simulink model "RO_Plantsimscape"  (R2020a)
settings: Solver=VariableStepAuto  StartTime=0.0  StopTime=100  RelTol=1e-3
libraries: sh_lib x108, fl_lib x76, nesl_utility x73, simulink x13
(part 2 of 4)

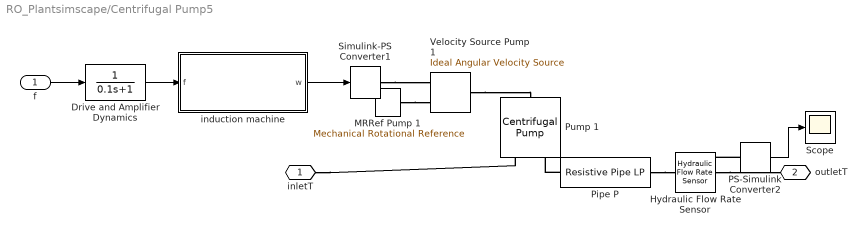
== system RO_Plantsimscape/Centrifugal Pump5 ==
  f : Inport
  Drive and Amplifier Dynamics : TransferFcn  Denominator=[0.1 1]
  Hydraulic Flow Rate Sensor : fl_lib/Hydraulic/Hydraulic Sensors/Hydraulic Flow Rate Sensor
  MRRef Pump 1 : fl_lib/Mechanical/Rotational Elements/Mechanical Rotational Reference
  PS-Simulink Converter2 : nesl_utility/PS-Simulink Converter  PhysicalDomain=network_engine_domain  SubClassName=ps_output  LeftPortType=input  RightPortType=output  PseudoPeriodic=off  Frequencies=[]  Unit=1  AffineConversion=off
  Pipe P : sh_lib/Low-Pressure Blocks/Resistive Pipe LP  cs_type=1  d_in=112.1660 mm  area=1e-04 m^2  D_h=0.0112 m  s_factor=64  length=8.1 m  length_ad=1 m  roughness=0.005 mm  Re_lam=2e+03  Re_turb=4e+03  elevation_A=45 m  elevation_B=45 m  g=9.80665 m/s^2  pressure_drop_specify=off  pressure_drop_priority=None  pressure_drop=0 Pa  pressure_drop_nominal_specify=off  pressure_drop_nominal_unit=Pa  pressure_drop_nominal_value=1  flow_rate_specify=off  flow_rate_priority=None  flow_rate=0 m^3/s  flow_rate_nominal_specify=off  flow_rate_nominal_unit=m^3/s  flow_rate_nominal_value=1
      settings: SourceProductBaseCode=SH  InternalSimscapePortConfiguration="{\"Bottom\":[],\"Left\":[{\"id\":\"A\",\"label\":\"A\",\"type\":\"foundation.hydraulic.hydraulic\"}],\"Right\":[{\"id\":\"B\",\"label\":\"B\",\"type\":\"foundation.hydraulic.hydraulic\"}],\"Top\":[]}"
  Pump 1 : sh_lib/Pumps and Motors/Centrifugal Pump  mdl_type=2  c_1=326.8 Pa/(kg/m^3)  c_2=3.104e+04 Pa*s/kg  c_3=1.097e+07 Pa*s^2/(kg*m^3)  c_4=2.136e+05 Pa*s^2/(kg*m^3)  c_f=0.8  design_del=130 lpm  ref_velocity=1.77e+03 rpm  ref_density=1000 kg/m^3  leak_resistance=1e+8 Pa/(m^3/s)  T_const=0.1 N*m  trq_press_coeff=1e-6 N*m/Pa  pump_del_1D="[0    0.0032    0.0063    0.0095    0.0126    0.0158] m^3/s"  press_diff_1D="[4.4851    4.3655    4.1413    3.7376    2.9901    1.7940] bar"  pump_del_power_1D="[0    0.0032    0.0063    0.0095    0.0126    0.0158] m^3/s"  power_1D="[0\t2116.60000000000\t3727.20000000000\t4734.30000000000\t5232.70000000000\t4360.90000000000] W"  pump_vel_2D="[  3.2e+03 3.3e+03 3.4e+03 3.5e+03 ] rpm"  pump_del_2D="[  0 50 100 150 200 250 300 350 ] lpm"  press_diff_2D="[  8.3 8.8 9.3 9.9 ; 7.8 8.3 8.8 9.4 ; 7.2 7.6 8.2 8.7 ; 6.5 7 7.5 8 ; 5.6 6.1 6.6 7.1 ; 4.7 5.2 5.7 6.2 ; 3.4 4 4.4 4.9 ; 2.3 2.7 3.4 3.6 ; ] bar"  pump_del_power_2D="[  0 50 100 150 200 250 300 350 ] lpm"  power_2D="[  1.223e+03 1.341e+03 1.467e+03 1.6e+03 ; 1.414e+03 1.551e+03 1.696e+03 1.85e+03 ; 1.636e+03 1.794e+03 1.962e+03 2.14e+03 ; 1.941e+03 2.129e+03 2.326e+03 2.54e+03 ; 2.224e+03 2.439e+03 2.66e+03 2.91e+03 ; 2.453e+03 2.691e+03 2.947e+03 3.21e+03 ; 2.757e+03 3.024e+03 3.307e+03 3.608e+03 ; 2.945e+03 3.23e+03 3.533e+03 3.854e+03 ; ] W"  omega_threshold=1e-9 rad/s  interp_method=2  extrap_method=1
      settings: SourceProductBaseCode=SH  InternalSimscapePortConfiguration="{\"Bottom\":[],\"Left\":[{\"id\":\"S\",\"label\":\"S\",\"type\":\"foundation.mechanical.rotational.rotational\"}],\"Right\":[{\"id\":\"P\",\"label\":\"P\",\"type\":\"foundation.hydraulic.hydraulic\"},{\"id\":\"T\",\"label\":\"T\",\"type\":\"foundation.hydraulic.hydraulic\"}],\"Top\":[]}"
  Scope : Scope
  Simulink-PS Converter1 : nesl_utility/Simulink-PS Converter  PhysicalDomain=network_engine_domain  SubClassName=ps_input  LeftPortType=input  RightPortType=output  PseudoPeriodic=off  Frequencies=[]  NoiseDistribution=none  NoiseParameters=[]  Unit=rpm  AffineConversion=off  FilteringAndDerivatives=zero  SimscapeFilterOrder=1  InputFilterTimeConstant=.001  UdotUserProvided=0
  Velocity Source Pump 1 : fl_lib/Mechanical/Mechanical Sources/Ideal Angular Velocity Source
  induction machine : Subsystem
  inletT : PMIOPort  Side=Left
  outletT : PMIOPort  Port=2  Side=Right
  wires:
  f/1 -> Drive and Amplifier Dynamics/1
  induction machine/1(w) -> Simulink-PS Converter1/1
  Drive and Amplifier Dynamics/1 -> induction machine/1(f)
  PS-Simulink Converter2/1 -> Scope/1
  connections:
  Velocity Source Pump 1/LConn1 -- Pump 1/LConn1
  MRRef Pump 1/LConn1 -- Velocity Source Pump 1/RConn2
  inletT/RConn1 -- Pump 1/RConn2
  Pipe P/LConn1 -- Pump 1/RConn1
  Simulink-PS Converter1/RConn1 -- Velocity Source Pump 1/RConn1
  Pipe P/RConn1 -- Hydraulic Flow Rate Sensor/LConn1
  Hydraulic Flow Rate Sensor/RConn2 -- outletT/RConn1
  PS-Simulink Converter2/LConn1 -- Hydraulic Flow Rate Sensor/RConn1

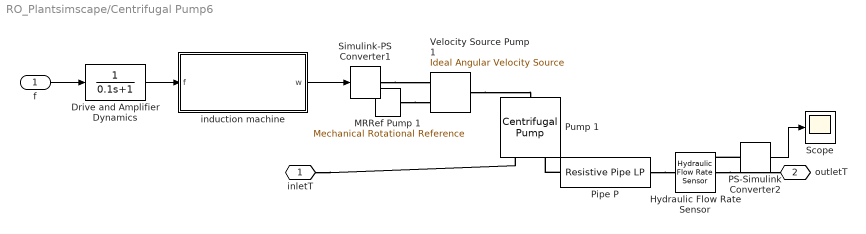
== system RO_Plantsimscape/Centrifugal Pump6 ==
  f : Inport
  Drive and Amplifier Dynamics : TransferFcn  Denominator=[0.1 1]
  Hydraulic Flow Rate Sensor : fl_lib/Hydraulic/Hydraulic Sensors/Hydraulic Flow Rate Sensor
  MRRef Pump 1 : fl_lib/Mechanical/Rotational Elements/Mechanical Rotational Reference
  PS-Simulink Converter2 : nesl_utility/PS-Simulink Converter  PhysicalDomain=network_engine_domain  SubClassName=ps_output  LeftPortType=input  RightPortType=output  PseudoPeriodic=off  Frequencies=[]  Unit=1  AffineConversion=off
  Pipe P : sh_lib/Low-Pressure Blocks/Resistive Pipe LP  cs_type=1  d_in=112.1660 mm  area=1e-04 m^2  D_h=0.0112 m  s_factor=64  length=8.1 m  length_ad=1 m  roughness=0.005 mm  Re_lam=2e+03  Re_turb=4e+03  elevation_A=45 m  elevation_B=45 m  g=9.80665 m/s^2  pressure_drop_specify=off  pressure_drop_priority=None  pressure_drop=0 Pa  pressure_drop_nominal_specify=off  pressure_drop_nominal_unit=Pa  pressure_drop_nominal_value=1  flow_rate_specify=off  flow_rate_priority=None  flow_rate=0 m^3/s  flow_rate_nominal_specify=off  flow_rate_nominal_unit=m^3/s  flow_rate_nominal_value=1
      settings: SourceProductBaseCode=SH  InternalSimscapePortConfiguration="{\"Bottom\":[],\"Left\":[{\"id\":\"A\",\"label\":\"A\",\"type\":\"foundation.hydraulic.hydraulic\"}],\"Right\":[{\"id\":\"B\",\"label\":\"B\",\"type\":\"foundation.hydraulic.hydraulic\"}],\"Top\":[]}"
  Pump 1 : sh_lib/Pumps and Motors/Centrifugal Pump  mdl_type=2  c_1=326.8 Pa/(kg/m^3)  c_2=3.104e+04 Pa*s/kg  c_3=1.097e+07 Pa*s^2/(kg*m^3)  c_4=2.136e+05 Pa*s^2/(kg*m^3)  c_f=0.8  design_del=130 lpm  ref_velocity=1.77e+03 rpm  ref_density=1000 kg/m^3  leak_resistance=1e+8 Pa/(m^3/s)  T_const=0.1 N*m  trq_press_coeff=1e-6 N*m/Pa  pump_del_1D="[0    0.0032    0.0063    0.0095    0.0126    0.0158] m^3/s"  press_diff_1D="[4.4851    4.3655    4.1413    3.7376    2.9901    1.7940] bar"  pump_del_power_1D="[0    0.0032    0.0063    0.0095    0.0126    0.0158] m^3/s"  power_1D="[0\t2116.60000000000\t3727.20000000000\t4734.30000000000\t5232.70000000000\t4360.90000000000] W"  pump_vel_2D="[  3.2e+03 3.3e+03 3.4e+03 3.5e+03 ] rpm"  pump_del_2D="[  0 50 100 150 200 250 300 350 ] lpm"  press_diff_2D="[  8.3 8.8 9.3 9.9 ; 7.8 8.3 8.8 9.4 ; 7.2 7.6 8.2 8.7 ; 6.5 7 7.5 8 ; 5.6 6.1 6.6 7.1 ; 4.7 5.2 5.7 6.2 ; 3.4 4 4.4 4.9 ; 2.3 2.7 3.4 3.6 ; ] bar"  pump_del_power_2D="[  0 50 100 150 200 250 300 350 ] lpm"  power_2D="[  1.223e+03 1.341e+03 1.467e+03 1.6e+03 ; 1.414e+03 1.551e+03 1.696e+03 1.85e+03 ; 1.636e+03 1.794e+03 1.962e+03 2.14e+03 ; 1.941e+03 2.129e+03 2.326e+03 2.54e+03 ; 2.224e+03 2.439e+03 2.66e+03 2.91e+03 ; 2.453e+03 2.691e+03 2.947e+03 3.21e+03 ; 2.757e+03 3.024e+03 3.307e+03 3.608e+03 ; 2.945e+03 3.23e+03 3.533e+03 3.854e+03 ; ] W"  omega_threshold=1e-9 rad/s  interp_method=2  extrap_method=1
      settings: SourceProductBaseCode=SH  InternalSimscapePortConfiguration="{\"Bottom\":[],\"Left\":[{\"id\":\"S\",\"label\":\"S\",\"type\":\"foundation.mechanical.rotational.rotational\"}],\"Right\":[{\"id\":\"P\",\"label\":\"P\",\"type\":\"foundation.hydraulic.hydraulic\"},{\"id\":\"T\",\"label\":\"T\",\"type\":\"foundation.hydraulic.hydraulic\"}],\"Top\":[]}"
  Scope : Scope
  Simulink-PS Converter1 : nesl_utility/Simulink-PS Converter  PhysicalDomain=network_engine_domain  SubClassName=ps_input  LeftPortType=input  RightPortType=output  PseudoPeriodic=off  Frequencies=[]  NoiseDistribution=none  NoiseParameters=[]  Unit=rpm  AffineConversion=off  FilteringAndDerivatives=zero  SimscapeFilterOrder=1  InputFilterTimeConstant=.001  UdotUserProvided=0
  Velocity Source Pump 1 : fl_lib/Mechanical/Mechanical Sources/Ideal Angular Velocity Source
  induction machine : Subsystem
  inletT : PMIOPort  Side=Left
  outletT : PMIOPort  Port=2  Side=Right
  wires:
  f/1 -> Drive and Amplifier Dynamics/1
  induction machine/1(w) -> Simulink-PS Converter1/1
  Drive and Amplifier Dynamics/1 -> induction machine/1(f)
  PS-Simulink Converter2/1 -> Scope/1
  connections:
  Velocity Source Pump 1/LConn1 -- Pump 1/LConn1
  MRRef Pump 1/LConn1 -- Velocity Source Pump 1/RConn2
  inletT/RConn1 -- Pump 1/RConn2
  Pipe P/LConn1 -- Pump 1/RConn1
  Simulink-PS Converter1/RConn1 -- Velocity Source Pump 1/RConn1
  Pipe P/RConn1 -- Hydraulic Flow Rate Sensor/LConn1
  Hydraulic Flow Rate Sensor/RConn2 -- outletT/RConn1
  PS-Simulink Converter2/LConn1 -- Hydraulic Flow Rate Sensor/RConn1

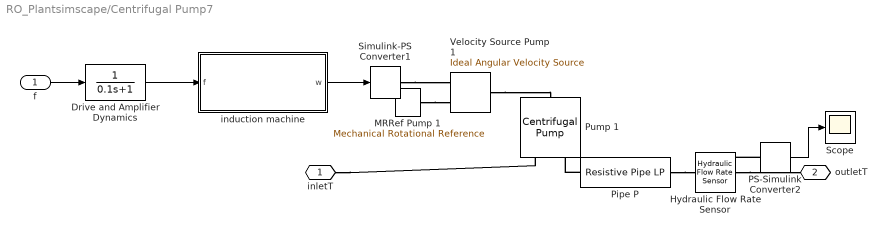
== system RO_Plantsimscape/Centrifugal Pump7 ==
  f : Inport
  Drive and Amplifier Dynamics : TransferFcn  Denominator=[0.1 1]
  Hydraulic Flow Rate Sensor : fl_lib/Hydraulic/Hydraulic Sensors/Hydraulic Flow Rate Sensor
  MRRef Pump 1 : fl_lib/Mechanical/Rotational Elements/Mechanical Rotational Reference
  PS-Simulink Converter2 : nesl_utility/PS-Simulink Converter  PhysicalDomain=network_engine_domain  SubClassName=ps_output  LeftPortType=input  RightPortType=output  PseudoPeriodic=off  Frequencies=[]  Unit=1  AffineConversion=off
  Pipe P : sh_lib/Low-Pressure Blocks/Resistive Pipe LP  cs_type=1  d_in=48 in  area=1e-04 m^2  D_h=0.0112 m  s_factor=7.15e-02  length=8.1 m  length_ad=1 m  roughness=0.005 mm  Re_lam=2e+03  Re_turb=4e+03  elevation_A=45 m  elevation_B=45 m  g=9.80665 m/s^2  pressure_drop_specify=off  pressure_drop_priority=None  pressure_drop=0 Pa  pressure_drop_nominal_specify=off  pressure_drop_nominal_unit=Pa  pressure_drop_nominal_value=1  flow_rate_specify=off  flow_rate_priority=None  flow_rate=0 m^3/s  flow_rate_nominal_specify=off  flow_rate_nominal_unit=m^3/s  flow_rate_nominal_value=1
      settings: SourceProductBaseCode=SH  InternalSimscapePortConfiguration="{\"Bottom\":[],\"Left\":[{\"id\":\"A\",\"label\":\"A\",\"type\":\"foundation.hydraulic.hydraulic\"}],\"Right\":[{\"id\":\"B\",\"label\":\"B\",\"type\":\"foundation.hydraulic.hydraulic\"}],\"Top\":[]}"
  Pump 1 : sh_lib/Pumps and Motors/Centrifugal Pump  mdl_type=1  c_1=3.268e+30 Pa/(kg/m^3)  c_2=3.104e+16 Pa*s/kg  c_3=1.097e+22 Pa*s^2/(kg*m^3)  c_4=2.136e+18 Pa*s^2/(kg*m^3)  c_f=0.8  design_del=2.5 m^3/s  ref_velocity=1.77e+03 rpm  ref_density=1000 kg/m^3  leak_resistance=1e+8 Pa/(m^3/s)  T_const=1000 N*m  trq_press_coeff=1e-6 N*m/Pa  pump_del_1D="[0    0.0032    0.0063    0.0095    0.0126    0.0158] m^3/s"  press_diff_1D="[4.4851    4.3655    4.1413    3.7376    2.9901    1.7940] bar"  pump_del_power_1D="[0    0.0032    0.0063    0.0095    0.0126    0.0158] m^3/s"  power_1D="[0\t2116.60000000000\t3727.20000000000\t4734.30000000000\t5232.70000000000\t4360.90000000000] W"  pump_vel_2D="[  3.2e+03 3.3e+03 3.4e+03 3.5e+03 ] rpm"  pump_del_2D="[  0 50 100 150 200 250 300 350 ] lpm"  press_diff_2D="[  8.3 8.8 9.3 9.9 ; 7.8 8.3 8.8 9.4 ; 7.2 7.6 8.2 8.7 ; 6.5 7 7.5 8 ; 5.6 6.1 6.6 7.1 ; 4.7 5.2 5.7 6.2 ; 3.4 4 4.4 4.9 ; 2.3 2.7 3.4 3.6 ; ] bar"  pump_del_power_2D="[  0 50 100 150 200 250 300 350 ] lpm"  power_2D="[  1.223e+03 1.341e+03 1.467e+03 1.6e+03 ; 1.414e+03 1.551e+03 1.696e+03 1.85e+03 ; 1.636e+03 1.794e+03 1.962e+03 2.14e+03 ; 1.941e+03 2.129e+03 2.326e+03 2.54e+03 ; 2.224e+03 2.439e+03 2.66e+03 2.91e+03 ; 2.453e+03 2.691e+03 2.947e+03 3.21e+03 ; 2.757e+03 3.024e+03 3.307e+03 3.608e+03 ; 2.945e+03 3.23e+03 3.533e+03 3.854e+03 ; ] W"  omega_threshold=1e-9 rad/s  interp_method=2  extrap_method=1
      settings: SourceProductBaseCode=SH  InternalSimscapePortConfiguration="{\"Bottom\":[],\"Left\":[{\"id\":\"S\",\"label\":\"S\",\"type\":\"foundation.mechanical.rotational.rotational\"}],\"Right\":[{\"id\":\"P\",\"label\":\"P\",\"type\":\"foundation.hydraulic.hydraulic\"},{\"id\":\"T\",\"label\":\"T\",\"type\":\"foundation.hydraulic.hydraulic\"}],\"Top\":[]}"
  Scope : Scope
  Simulink-PS Converter1 : nesl_utility/Simulink-PS Converter  PhysicalDomain=network_engine_domain  SubClassName=ps_input  LeftPortType=input  RightPortType=output  PseudoPeriodic=off  Frequencies=[]  NoiseDistribution=none  NoiseParameters=[]  Unit=rpm  AffineConversion=off  FilteringAndDerivatives=zero  SimscapeFilterOrder=1  InputFilterTimeConstant=.001  UdotUserProvided=0
  Velocity Source Pump 1 : fl_lib/Mechanical/Mechanical Sources/Ideal Angular Velocity Source
  induction machine : Subsystem
  inletT : PMIOPort  Side=Left
  outletT : PMIOPort  Port=2  Side=Right
  wires:
  f/1 -> Drive and Amplifier Dynamics/1
  induction machine/1(w) -> Simulink-PS Converter1/1
  Drive and Amplifier Dynamics/1 -> induction machine/1(f)
  PS-Simulink Converter2/1 -> Scope/1
  connections:
  Velocity Source Pump 1/LConn1 -- Pump 1/LConn1
  MRRef Pump 1/LConn1 -- Velocity Source Pump 1/RConn2
  inletT/RConn1 -- Pump 1/RConn2
  Pipe P/LConn1 -- Pump 1/RConn1
  Simulink-PS Converter1/RConn1 -- Velocity Source Pump 1/RConn1
  Pipe P/RConn1 -- Hydraulic Flow Rate Sensor/LConn1
  Hydraulic Flow Rate Sensor/RConn2 -- outletT/RConn1
  PS-Simulink Converter2/LConn1 -- Hydraulic Flow Rate Sensor/RConn1

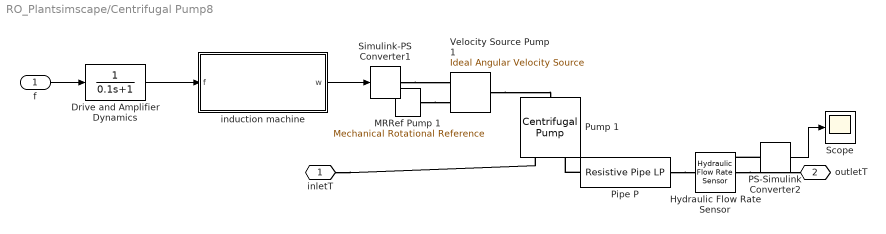
== system RO_Plantsimscape/Centrifugal Pump8 ==
  f : Inport
  Drive and Amplifier Dynamics : TransferFcn  Denominator=[0.1 1]
  Hydraulic Flow Rate Sensor : fl_lib/Hydraulic/Hydraulic Sensors/Hydraulic Flow Rate Sensor
  MRRef Pump 1 : fl_lib/Mechanical/Rotational Elements/Mechanical Rotational Reference
  PS-Simulink Converter2 : nesl_utility/PS-Simulink Converter  PhysicalDomain=network_engine_domain  SubClassName=ps_output  LeftPortType=input  RightPortType=output  PseudoPeriodic=off  Frequencies=[]  Unit=1  AffineConversion=off
  Pipe P : sh_lib/Low-Pressure Blocks/Resistive Pipe LP  cs_type=1  d_in=112.1660 mm  area=1e-04 m^2  D_h=0.0112 m  s_factor=64  length=8.1 m  length_ad=1 m  roughness=0.005 mm  Re_lam=2e+03  Re_turb=4e+03  elevation_A=45 m  elevation_B=45 m  g=9.80665 m/s^2  pressure_drop_specify=off  pressure_drop_priority=None  pressure_drop=0 Pa  pressure_drop_nominal_specify=off  pressure_drop_nominal_unit=Pa  pressure_drop_nominal_value=1  flow_rate_specify=off  flow_rate_priority=None  flow_rate=0 m^3/s  flow_rate_nominal_specify=off  flow_rate_nominal_unit=m^3/s  flow_rate_nominal_value=1
      settings: SourceProductBaseCode=SH  InternalSimscapePortConfiguration="{\"Bottom\":[],\"Left\":[{\"id\":\"A\",\"label\":\"A\",\"type\":\"foundation.hydraulic.hydraulic\"}],\"Right\":[{\"id\":\"B\",\"label\":\"B\",\"type\":\"foundation.hydraulic.hydraulic\"}],\"Top\":[]}"
  Pump 1 : sh_lib/Pumps and Motors/Centrifugal Pump  mdl_type=2  c_1=326.8 Pa/(kg/m^3)  c_2=3.104e+04 Pa*s/kg  c_3=1.097e+07 Pa*s^2/(kg*m^3)  c_4=2.136e+05 Pa*s^2/(kg*m^3)  c_f=0.8  design_del=130 lpm  ref_velocity=1.77e+03 rpm  ref_density=1000 kg/m^3  leak_resistance=1e+8 Pa/(m^3/s)  T_const=0.1 N*m  trq_press_coeff=1e-6 N*m/Pa  pump_del_1D="[0    0.0032    0.0063    0.0095    0.0126    0.0158] m^3/s"  press_diff_1D="[4.4851    4.3655    4.1413    3.7376    2.9901    1.7940] bar"  pump_del_power_1D="[0    0.0032    0.0063    0.0095    0.0126    0.0158] m^3/s"  power_1D="[0\t2116.60000000000\t3727.20000000000\t4734.30000000000\t5232.70000000000\t4360.90000000000] W"  pump_vel_2D="[  3.2e+03 3.3e+03 3.4e+03 3.5e+03 ] rpm"  pump_del_2D="[  0 50 100 150 200 250 300 350 ] lpm"  press_diff_2D="[  8.3 8.8 9.3 9.9 ; 7.8 8.3 8.8 9.4 ; 7.2 7.6 8.2 8.7 ; 6.5 7 7.5 8 ; 5.6 6.1 6.6 7.1 ; 4.7 5.2 5.7 6.2 ; 3.4 4 4.4 4.9 ; 2.3 2.7 3.4 3.6 ; ] bar"  pump_del_power_2D="[  0 50 100 150 200 250 300 350 ] lpm"  power_2D="[  1.223e+03 1.341e+03 1.467e+03 1.6e+03 ; 1.414e+03 1.551e+03 1.696e+03 1.85e+03 ; 1.636e+03 1.794e+03 1.962e+03 2.14e+03 ; 1.941e+03 2.129e+03 2.326e+03 2.54e+03 ; 2.224e+03 2.439e+03 2.66e+03 2.91e+03 ; 2.453e+03 2.691e+03 2.947e+03 3.21e+03 ; 2.757e+03 3.024e+03 3.307e+03 3.608e+03 ; 2.945e+03 3.23e+03 3.533e+03 3.854e+03 ; ] W"  omega_threshold=1e-9 rad/s  interp_method=2  extrap_method=1
      settings: SourceProductBaseCode=SH  InternalSimscapePortConfiguration="{\"Bottom\":[],\"Left\":[{\"id\":\"S\",\"label\":\"S\",\"type\":\"foundation.mechanical.rotational.rotational\"}],\"Right\":[{\"id\":\"P\",\"label\":\"P\",\"type\":\"foundation.hydraulic.hydraulic\"},{\"id\":\"T\",\"label\":\"T\",\"type\":\"foundation.hydraulic.hydraulic\"}],\"Top\":[]}"
  Scope : Scope
  Simulink-PS Converter1 : nesl_utility/Simulink-PS Converter  PhysicalDomain=network_engine_domain  SubClassName=ps_input  LeftPortType=input  RightPortType=output  PseudoPeriodic=off  Frequencies=[]  NoiseDistribution=none  NoiseParameters=[]  Unit=rpm  AffineConversion=off  FilteringAndDerivatives=zero  SimscapeFilterOrder=1  InputFilterTimeConstant=.001  UdotUserProvided=0
  Velocity Source Pump 1 : fl_lib/Mechanical/Mechanical Sources/Ideal Angular Velocity Source
  induction machine : Subsystem
  inletT : PMIOPort  Side=Left
  outletT : PMIOPort  Port=2  Side=Right
  wires:
  f/1 -> Drive and Amplifier Dynamics/1
  induction machine/1(w) -> Simulink-PS Converter1/1
  Drive and Amplifier Dynamics/1 -> induction machine/1(f)
  PS-Simulink Converter2/1 -> Scope/1
  connections:
  Velocity Source Pump 1/LConn1 -- Pump 1/LConn1
  MRRef Pump 1/LConn1 -- Velocity Source Pump 1/RConn2
  inletT/RConn1 -- Pump 1/RConn2
  Pipe P/LConn1 -- Pump 1/RConn1
  Simulink-PS Converter1/RConn1 -- Velocity Source Pump 1/RConn1
  Pipe P/RConn1 -- Hydraulic Flow Rate Sensor/LConn1
  Hydraulic Flow Rate Sensor/RConn2 -- outletT/RConn1
  PS-Simulink Converter2/LConn1 -- Hydraulic Flow Rate Sensor/RConn1

== system RO_Plantsimscape/D1 ==
  Local Resistance : sh_lib/Local Hydraulic Resistances/Local Resistance  area=1e-4 m^2  mdl_type=1  kp_d=2  kp_r=2  lam_spec=1  B_lam=0.999  Re_cr=150  Re_vec=[-4000, -3000, -2000, -1000, -500, -200, -100, -50, -40, -30, -20, -15, -10, 10, 20, 30, 40, 50, 100, 200, 500, 1000, 2000, 4000, 5000, 10000]  loss_coeff_vec=[.25, .3, .65, .9, .65, .75, .9, 1.15, 1.35, 1.65, 2.3, 2.8, 3.1, 5, 2.7, 1.8, 1.46, 1.3, .9, .65, .42, .3, .2, .4, .42, .25]  interp_method=2  extrap_method=2  flow_rate_threshold=1e-6 m^3/s  flow_rate_specify=off  flow_rate_priority=None  flow_rate=0 m^3/s  flow_rate_nominal_specify=off  flow_rate_nominal_unit=m^3/s  flow_rate_nominal_value=1  pressure_drop_specify=off  pressure_drop_priority=None  pressure_drop=0 Pa  pressure_drop_nominal_specify=off  pressure_drop_nominal_unit=Pa  pressure_drop_nominal_value=1
      settings: SourceProductBaseCode=SH  InternalSimscapePortConfiguration="{\"Bottom\":[],\"Left\":[{\"id\":\"A\",\"label\":\"A\",\"type\":\"foundation.hydraulic.hydraulic\"}],\"Right\":[{\"id\":\"B\",\"label\":\"B\",\"type\":\"foundation.hydraulic.hydraulic\"}],\"Top\":[]}"
  Mineral Tank : sh_lib/Hydraulic Utilities/Reservoir  press=1 atm  init_volume=0 m^3  ret_diam=0.02 m  loss_coeff=1
      settings: SourceProductBaseCode=SH  InternalSimscapePortConfiguration="{\"Bottom\":[],\"Left\":[{\"id\":\"V\",\"label\":\"V\",\"type\":\"output\"},{\"id\":\"P\",\"label\":\"P\",\"type\":\"foundation.hydraulic.hydraulic\"},{\"id\":\"R\",\"label\":\"R\",\"type\":\"foundation.hydraulic.hydraulic\"}],\"Right\":[],\"Top\":[]}"
  IN : PMIOPort  Side=Left
  OUT : PMIOPort  Port=2  Side=Right
  connections:
  Mineral Tank/LConn2 -- IN/RConn1
  Mineral Tank/LConn3 -- Local Resistance/LConn1
  OUT/RConn1 -- Local Resistance/RConn1

== system RO_Plantsimscape/FC1 ==
  Hydraulic Flow Rate Sensor : fl_lib/Hydraulic/Hydraulic Sensors/Hydraulic Flow Rate Sensor
  Local Resistance : sh_lib/Local Hydraulic Resistances/Local Resistance  area=1e-4 m^2  mdl_type=1  kp_d=2  kp_r=2  lam_spec=1  B_lam=0.999  Re_cr=150  Re_vec=[-4000, -3000, -2000, -1000, -500, -200, -100, -50, -40, -30, -20, -15, -10, 10, 20, 30, 40, 50, 100, 200, 500, 1000, 2000, 4000, 5000, 10000]  loss_coeff_vec=[.25, .3, .65, .9, .65, .75, .9, 1.15, 1.35, 1.65, 2.3, 2.8, 3.1, 5, 2.7, 1.8, 1.46, 1.3, .9, .65, .42, .3, .2, .4, .42, .25]  interp_method=2  extrap_method=2  flow_rate_threshold=1e-6 m^3/s  flow_rate_specify=on  flow_rate_priority=None  flow_rate=4 gpm  flow_rate_nominal_specify=off  flow_rate_nominal_unit=m^3/s  flow_rate_nominal_value=1  pressure_drop_specify=on  pressure_drop_priority=None  pressure_drop=25 psi  pressure_drop_nominal_specify=off  pressure_drop_nominal_unit=Pa  pressure_drop_nominal_value=1
      settings: SourceProductBaseCode=SH  InternalSimscapePortConfiguration="{\"Bottom\":[],\"Left\":[{\"id\":\"A\",\"label\":\"A\",\"type\":\"foundation.hydraulic.hydraulic\"}],\"Right\":[{\"id\":\"B\",\"label\":\"B\",\"type\":\"foundation.hydraulic.hydraulic\"}],\"Top\":[]}"
  PS-Simulink Converter2 : nesl_utility/PS-Simulink Converter  PhysicalDomain=network_engine_domain  SubClassName=ps_output  LeftPortType=input  RightPortType=output  PseudoPeriodic=off  Frequencies=[]  Unit=1  AffineConversion=off
  Resistive Pipe LP : sh_lib/Low-Pressure Blocks/Resistive Pipe LP  cs_type=1  d_in=0.01 m  area=1e-4 m^2  D_h=1.12e-2 m  s_factor=64  length=5 m  length_ad=1 m  roughness=15e-6 m  Re_lam=2000  Re_turb=4000  elevation_A=0 m  elevation_B=0 m  g=9.80665 m/s^2  pressure_drop_specify=off  pressure_drop_priority=None  pressure_drop=0 Pa  pressure_drop_nominal_specify=off  pressure_drop_nominal_unit=Pa  pressure_drop_nominal_value=1  flow_rate_specify=off  flow_rate_priority=None  flow_rate=0 m^3/s  flow_rate_nominal_specify=off  flow_rate_nominal_unit=m^3/s  flow_rate_nominal_value=1
      settings: SourceProductBaseCode=SH  InternalSimscapePortConfiguration="{\"Bottom\":[],\"Left\":[{\"id\":\"A\",\"label\":\"A\",\"type\":\"foundation.hydraulic.hydraulic\"}],\"Right\":[{\"id\":\"B\",\"label\":\"B\",\"type\":\"foundation.hydraulic.hydraulic\"}],\"Top\":[]}"
  Scope : Scope
  IN : PMIOPort  Side=Left
  OUT : PMIOPort  Port=2  Side=Right
  wires:
  PS-Simulink Converter2/1 -> Scope/1
  connections:
  IN/RConn1 -- Local Resistance/LConn1
  Hydraulic Flow Rate Sensor/LConn1 -- Resistive Pipe LP/RConn1
  Hydraulic Flow Rate Sensor/RConn2 -- OUT/RConn1
  Hydraulic Flow Rate Sensor/RConn1 -- PS-Simulink Converter2/LConn1
  Local Resistance/RConn1 -- Resistive Pipe LP/LConn1

== system RO_Plantsimscape/FC2 ==
  Hydraulic Flow Rate Sensor : fl_lib/Hydraulic/Hydraulic Sensors/Hydraulic Flow Rate Sensor
  Local Resistance : sh_lib/Local Hydraulic Resistances/Local Resistance  area=1e-4 m^2  mdl_type=1  kp_d=2  kp_r=2  lam_spec=1  B_lam=0.999  Re_cr=150  Re_vec=[-4000, -3000, -2000, -1000, -500, -200, -100, -50, -40, -30, -20, -15, -10, 10, 20, 30, 40, 50, 100, 200, 500, 1000, 2000, 4000, 5000, 10000]  loss_coeff_vec=[.25, .3, .65, .9, .65, .75, .9, 1.15, 1.35, 1.65, 2.3, 2.8, 3.1, 5, 2.7, 1.8, 1.46, 1.3, .9, .65, .42, .3, .2, .4, .42, .25]  interp_method=2  extrap_method=2  flow_rate_threshold=1e-6 m^3/s  flow_rate_specify=on  flow_rate_priority=None  flow_rate=4 gpm  flow_rate_nominal_specify=off  flow_rate_nominal_unit=m^3/s  flow_rate_nominal_value=1  pressure_drop_specify=on  pressure_drop_priority=None  pressure_drop=25 psi  pressure_drop_nominal_specify=off  pressure_drop_nominal_unit=Pa  pressure_drop_nominal_value=1
      settings: SourceProductBaseCode=SH  InternalSimscapePortConfiguration="{\"Bottom\":[],\"Left\":[{\"id\":\"A\",\"label\":\"A\",\"type\":\"foundation.hydraulic.hydraulic\"}],\"Right\":[{\"id\":\"B\",\"label\":\"B\",\"type\":\"foundation.hydraulic.hydraulic\"}],\"Top\":[]}"
  PS-Simulink Converter2 : nesl_utility/PS-Simulink Converter  PhysicalDomain=network_engine_domain  SubClassName=ps_output  LeftPortType=input  RightPortType=output  PseudoPeriodic=off  Frequencies=[]  Unit=1  AffineConversion=off
  Resistive Pipe LP : sh_lib/Low-Pressure Blocks/Resistive Pipe LP  cs_type=1  d_in=0.01 m  area=1e-4 m^2  D_h=1.12e-2 m  s_factor=64  length=5 m  length_ad=1 m  roughness=15e-6 m  Re_lam=2000  Re_turb=4000  elevation_A=0 m  elevation_B=0 m  g=9.80665 m/s^2  pressure_drop_specify=off  pressure_drop_priority=None  pressure_drop=0 Pa  pressure_drop_nominal_specify=off  pressure_drop_nominal_unit=Pa  pressure_drop_nominal_value=1  flow_rate_specify=off  flow_rate_priority=None  flow_rate=0 m^3/s  flow_rate_nominal_specify=off  flow_rate_nominal_unit=m^3/s  flow_rate_nominal_value=1
      settings: SourceProductBaseCode=SH  InternalSimscapePortConfiguration="{\"Bottom\":[],\"Left\":[{\"id\":\"A\",\"label\":\"A\",\"type\":\"foundation.hydraulic.hydraulic\"}],\"Right\":[{\"id\":\"B\",\"label\":\"B\",\"type\":\"foundation.hydraulic.hydraulic\"}],\"Top\":[]}"
  Scope : Scope
  IN : PMIOPort  Side=Left
  OUT : PMIOPort  Port=2  Side=Right
  wires:
  PS-Simulink Converter2/1 -> Scope/1
  connections:
  Hydraulic Flow Rate Sensor/LConn1 -- Resistive Pipe LP/RConn1
  Hydraulic Flow Rate Sensor/RConn2 -- OUT/RConn1
  Hydraulic Flow Rate Sensor/RConn1 -- PS-Simulink Converter2/LConn1
  Local Resistance/LConn1 -- IN/RConn1
  Local Resistance/RConn1 -- Resistive Pipe LP/LConn1

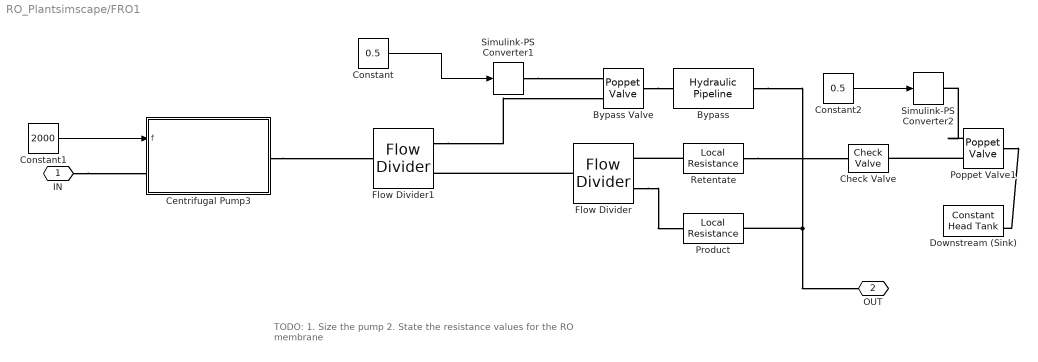
== system RO_Plantsimscape/FRO1 ==
  note: TODO:
      | 1. Size the pump
      | 2. State the resistance values for the RO membrane
  Bypass : sh_lib/Pipelines/Hydraulic Pipeline  cs_type=1  d_in=0.01 m  area=1e-4 m^2  D_h=1.12e-2 m  s_factor=64  length=5 m  length_ad=1 m  roughness=15e-6 m  Re_lam=2000  Re_turb=4000  wall_type=1  pr_r_coef=2e-12 m/Pa  time_const=0.01 s  k_sh=1.4  initial_pressure=0 Pa
      settings: SourceProductBaseCode=SH  InternalSimscapePortConfiguration="{\"Bottom\":[],\"Left\":[{\"id\":\"A\",\"label\":\"A\",\"type\":\"foundation.hydraulic.hydraulic\"}],\"Right\":[{\"id\":\"B\",\"label\":\"B\",\"type\":\"foundation.hydraulic.hydraulic\"}],\"Top\":[]}"
  Bypass Valve : sh_lib/Valves/Flow Control Valves/Poppet Valve  d_stem=0.01 m  cone_angle=120 deg  x_0=0 m  C_d=0.65  A_leak=1e-12 m^2  lam_spec=1  B_lam=0.999  Re_cr=10
      settings: SourceProductBaseCode=SH  InternalSimscapePortConfiguration="{\"Bottom\":[],\"Left\":[{\"id\":\"S\",\"label\":\"S\",\"type\":\"input\"},{\"id\":\"A\",\"label\":\"A\",\"type\":\"foundation.hydraulic.hydraulic\"}],\"Right\":[{\"id\":\"B\",\"label\":\"B\",\"type\":\"foundation.hydraulic.hydraulic\"}],\"Top\":[]}"
  Centrifugal Pump3 : Subsystem
      mask Display: image('$imagefile'); % Use "Edit Image" on toolstrip to change.
  Check Valve : sh_lib/Valves/Directional Valves/Check Valve  area_max=1e-4 m^2  pres_crack=0.3e5 Pa  pres_max=1.2e5 Pa  C_d=0.7  A_leak=1e-12 m^2  lam_spec=1  B_lam=0.999  Re_cr=12  dynamic=0  tau=0.1 s  area_init=1e-12 m^2
      settings: SourceProductBaseCode=SH  InternalSimscapePortConfiguration="{\"Bottom\":[],\"Left\":[{\"id\":\"A\",\"label\":\"A\",\"type\":\"foundation.hydraulic.hydraulic\"}],\"Right\":[{\"id\":\"B\",\"label\":\"B\",\"type\":\"foundation.hydraulic.hydraulic\"}],\"Top\":[]}"
  Constant : Constant  Value=0.5
  Constant1 : Constant  Value=2000
  Constant2 : Constant  Value=0.5
  Downstream (Sink) : sh_lib/Low-Pressure Blocks/Constant Head Tank  press=0 Pa  fluid_level=0 m  pipe_diam=0.02 m  loss_coeff=1.2  g=9.80665 m/s^2  volume_specify=on  volume_priority=High  volume=0 m^3  volume_nominal_specify=off  volume_nominal_unit=m^3  volume_nominal_value=1
      settings: SourceProductBaseCode=SH  InternalSimscapePortConfiguration="{\"Bottom\":[],\"Left\":[],\"Right\":[{\"id\":\"V\",\"label\":\"V\",\"type\":\"output\"},{\"id\":\"T\",\"label\":\"T\",\"type\":\"foundation.hydraulic.hydraulic\"}],\"Top\":[]}"
  Flow Divider : sh_lib/Valves/Flow Control Valves/Flow Divider  area_A=1e-4 m^2  area_B=1e-4 m^2  C_d_A=0.7  C_d_B=0.7  lam_spec=2  B_lam_A=0.999  B_lam_B=0.999  Re_cr_A=2300  Re_cr_B=2300  orifice_d=0.005 m  orifice_numb=4  C_d_or=0.65  init_A=0.0025 m  init_B=0.0025 m  leak_area=1e-9 m^2  lam_spec_or=1  B_lam_or_A=0.999  B_lam_or_B=0.999  Re_cr_or_A=10  Re_cr_or_B=10  area_sc=1.6e-4 m^2  stroke=0.005 m  spring_rate=1e3 N/m  damping=150 N/(m/s)  stop_coefficient=1e12 s*N/m^2
      settings: SourceProductBaseCode=SH  InternalSimscapePortConfiguration="{\"Bottom\":[],\"Left\":[{\"id\":\"P\",\"label\":\"P\",\"type\":\"foundation.hydraulic.hydraulic\"}],\"Right\":[{\"id\":\"A\",\"label\":\"A\",\"type\":\"foundation.hydraulic.hydraulic\"},{\"id\":\"B\",\"label\":\"B\",\"type\":\"foundation.hydraulic.hydraulic\"}],\"Top\":[]}"
  Flow Divider1 : sh_lib/Valves/Flow Control Valves/Flow Divider  area_A=1e-4 m^2  area_B=1e-4 m^2  C_d_A=0.7  C_d_B=0.7  lam_spec=2  B_lam_A=0.999  B_lam_B=0.999  Re_cr_A=2300  Re_cr_B=2300  orifice_d=0.005 m  orifice_numb=4  C_d_or=0.65  init_A=0.0025 m  init_B=0.0025 m  leak_area=1e-9 m^2  lam_spec_or=1  B_lam_or_A=0.999  B_lam_or_B=0.999  Re_cr_or_A=10  Re_cr_or_B=10  area_sc=1.6e-4 m^2  stroke=0.005 m  spring_rate=1e3 N/m  damping=150 N/(m/s)  stop_coefficient=1e12 s*N/m^2
      settings: SourceProductBaseCode=SH  InternalSimscapePortConfiguration="{\"Bottom\":[],\"Left\":[{\"id\":\"P\",\"label\":\"P\",\"type\":\"foundation.hydraulic.hydraulic\"}],\"Right\":[{\"id\":\"A\",\"label\":\"A\",\"type\":\"foundation.hydraulic.hydraulic\"},{\"id\":\"B\",\"label\":\"B\",\"type\":\"foundation.hydraulic.hydraulic\"}],\"Top\":[]}"
  Poppet Valve1 : sh_lib/Valves/Flow Control Valves/Poppet Valve  d_stem=0.01 m  cone_angle=120 deg  x_0=0 m  C_d=0.65  A_leak=1e-12 m^2  lam_spec=1  B_lam=0.999  Re_cr=10
      settings: SourceProductBaseCode=SH  InternalSimscapePortConfiguration="{\"Bottom\":[],\"Left\":[{\"id\":\"S\",\"label\":\"S\",\"type\":\"input\"},{\"id\":\"A\",\"label\":\"A\",\"type\":\"foundation.hydraulic.hydraulic\"}],\"Right\":[{\"id\":\"B\",\"label\":\"B\",\"type\":\"foundation.hydraulic.hydraulic\"}],\"Top\":[]}"
  Product : sh_lib/Local Hydraulic Resistances/Local Resistance  area=1e-4 m^2  mdl_type=1  kp_d=2  kp_r=2  lam_spec=2  B_lam=0.999  Re_cr=2300  Re_vec=[-4000, -3000, -2000, -1000, -500, -200, -100, -50, -40, -30, -20, -15, -10, 10, 20, 30, 40, 50, 100, 200, 500, 1000, 2000, 4000, 5000, 10000]  loss_coeff_vec=[.25, .3, .65, .9, .65, .75, .9, 1.15, 1.35, 1.65, 2.3, 2.8, 3.1, 5, 2.7, 1.8, 1.46, 1.3, .9, .65, .42, .3, .2, .4, .42, .25]  interp_method=2  extrap_method=2  flow_rate_threshold=1e-6 m^3/s  flow_rate_specify=off  flow_rate_priority=None  flow_rate=0 m^3/s  flow_rate_nominal_specify=off  flow_rate_nominal_unit=m^3/s  flow_rate_nominal_value=1  pressure_drop_specify=on  pressure_drop_priority=None  pressure_drop=10 psi  pressure_drop_nominal_specify=off  pressure_drop_nominal_unit=Pa  pressure_drop_nominal_value=1
      settings: SourceProductBaseCode=SH  InternalSimscapePortConfiguration="{\"Bottom\":[],\"Left\":[{\"id\":\"A\",\"label\":\"A\",\"type\":\"foundation.hydraulic.hydraulic\"}],\"Right\":[{\"id\":\"B\",\"label\":\"B\",\"type\":\"foundation.hydraulic.hydraulic\"}],\"Top\":[]}"
  Retentate : sh_lib/Local Hydraulic Resistances/Local Resistance  area=1e-4 m^2  mdl_type=1  kp_d=2  kp_r=2  lam_spec=2  B_lam=0.999  Re_cr=2300  Re_vec=[-4000, -3000, -2000, -1000, -500, -200, -100, -50, -40, -30, -20, -15, -10, 10, 20, 30, 40, 50, 100, 200, 500, 1000, 2000, 4000, 5000, 10000]  loss_coeff_vec=[.25, .3, .65, .9, .65, .75, .9, 1.15, 1.35, 1.65, 2.3, 2.8, 3.1, 5, 2.7, 1.8, 1.46, 1.3, .9, .65, .42, .3, .2, .4, .42, .25]  interp_method=2  extrap_method=2  flow_rate_threshold=1e-6 m^3/s  flow_rate_specify=off  flow_rate_priority=None  flow_rate=0 m^3/s  flow_rate_nominal_specify=off  flow_rate_nominal_unit=m^3/s  flow_rate_nominal_value=1  pressure_drop_specify=on  pressure_drop_priority=None  pressure_drop=10 psi  pressure_drop_nominal_specify=off  pressure_drop_nominal_unit=Pa  pressure_drop_nominal_value=1
      settings: SourceProductBaseCode=SH  InternalSimscapePortConfiguration="{\"Bottom\":[],\"Left\":[{\"id\":\"A\",\"label\":\"A\",\"type\":\"foundation.hydraulic.hydraulic\"}],\"Right\":[{\"id\":\"B\",\"label\":\"B\",\"type\":\"foundation.hydraulic.hydraulic\"}],\"Top\":[]}"
  Simulink-PS Converter1 : nesl_utility/Simulink-PS Converter  PhysicalDomain=network_engine_domain  SubClassName=ps_input  LeftPortType=input  RightPortType=output  PseudoPeriodic=off  Frequencies=[]  NoiseDistribution=none  NoiseParameters=[]  Unit=1  AffineConversion=off  FilteringAndDerivatives=zero  SimscapeFilterOrder=1  InputFilterTimeConstant=.001  UdotUserProvided=0
  Simulink-PS Converter2 : nesl_utility/Simulink-PS Converter  PhysicalDomain=network_engine_domain  SubClassName=ps_input  LeftPortType=input  RightPortType=output  PseudoPeriodic=off  Frequencies=[]  NoiseDistribution=none  NoiseParameters=[]  Unit=1  AffineConversion=off  FilteringAndDerivatives=zero  SimscapeFilterOrder=1  InputFilterTimeConstant=.001  UdotUserProvided=0
  IN : PMIOPort  Side=Left
  OUT : PMIOPort  Port=2  Side=Right
  wires:
  Constant/1 -> Simulink-PS Converter1/1
  Constant1/1 -> Centrifugal Pump3/1(f)
  Constant2/1 -> Simulink-PS Converter2/1
  connections:
  Retentate/LConn1 -- Flow Divider/RConn1
  Flow Divider/RConn2 -- Product/LConn1
  Flow Divider/LConn1 -- Flow Divider1/RConn2
  Flow Divider1/RConn1 -- Bypass Valve/LConn2
  Centrifugal Pump3/RConn1 -- Flow Divider1/LConn1
  IN/RConn1 -- Centrifugal Pump3/LConn1
  Simulink-PS Converter1/RConn1 -- Bypass Valve/LConn1
  Bypass Valve/RConn1 -- Bypass/LConn1
  Retentate/RConn1 -- Check Valve/RConn1
  Poppet Valve1/LConn1 -- Simulink-PS Converter2/RConn1
  Poppet Valve1/RConn1 -- Downstream (Sink)/RConn2
  Poppet Valve1/LConn2 -- Check Valve/LConn1
  Product/RConn1 -- Bypass/RConn1 -- OUT/RConn1

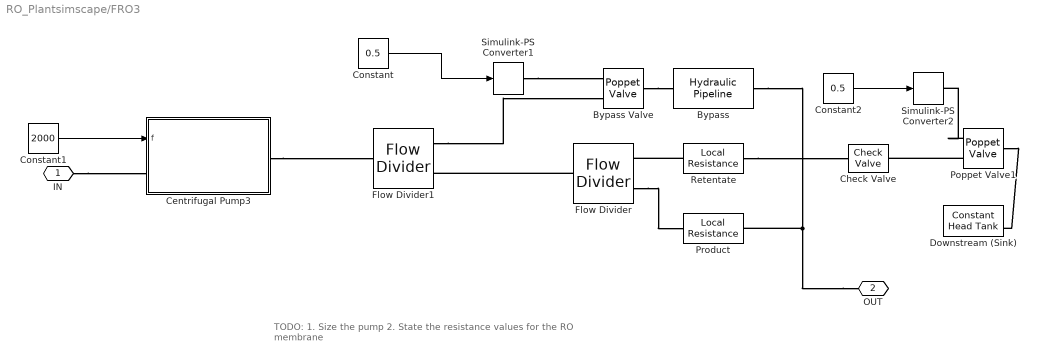
== system RO_Plantsimscape/FRO3 ==
  note: TODO:
      | 1. Size the pump
      | 2. State the resistance values for the RO membrane
  Bypass : sh_lib/Pipelines/Hydraulic Pipeline  cs_type=1  d_in=0.01 m  area=1e-4 m^2  D_h=1.12e-2 m  s_factor=64  length=5 m  length_ad=1 m  roughness=15e-6 m  Re_lam=2000  Re_turb=4000  wall_type=1  pr_r_coef=2e-12 m/Pa  time_const=0.01 s  k_sh=1.4  initial_pressure=0 Pa
      settings: SourceProductBaseCode=SH  InternalSimscapePortConfiguration="{\"Bottom\":[],\"Left\":[{\"id\":\"A\",\"label\":\"A\",\"type\":\"foundation.hydraulic.hydraulic\"}],\"Right\":[{\"id\":\"B\",\"label\":\"B\",\"type\":\"foundation.hydraulic.hydraulic\"}],\"Top\":[]}"
  Bypass Valve : sh_lib/Valves/Flow Control Valves/Poppet Valve  d_stem=0.01 m  cone_angle=120 deg  x_0=0 m  C_d=0.65  A_leak=1e-12 m^2  lam_spec=1  B_lam=0.999  Re_cr=10
      settings: SourceProductBaseCode=SH  InternalSimscapePortConfiguration="{\"Bottom\":[],\"Left\":[{\"id\":\"S\",\"label\":\"S\",\"type\":\"input\"},{\"id\":\"A\",\"label\":\"A\",\"type\":\"foundation.hydraulic.hydraulic\"}],\"Right\":[{\"id\":\"B\",\"label\":\"B\",\"type\":\"foundation.hydraulic.hydraulic\"}],\"Top\":[]}"
  Centrifugal Pump3 : Subsystem
      mask Display: image('$imagefile'); % Use "Edit Image" on toolstrip to change.
  Check Valve : sh_lib/Valves/Directional Valves/Check Valve  area_max=1e-4 m^2  pres_crack=0.3e5 Pa  pres_max=1.2e5 Pa  C_d=0.7  A_leak=1e-12 m^2  lam_spec=1  B_lam=0.999  Re_cr=12  dynamic=0  tau=0.1 s  area_init=1e-12 m^2
      settings: SourceProductBaseCode=SH  InternalSimscapePortConfiguration="{\"Bottom\":[],\"Left\":[{\"id\":\"A\",\"label\":\"A\",\"type\":\"foundation.hydraulic.hydraulic\"}],\"Right\":[{\"id\":\"B\",\"label\":\"B\",\"type\":\"foundation.hydraulic.hydraulic\"}],\"Top\":[]}"
  Constant : Constant  Value=0.5
  Constant1 : Constant  Value=2000
  Constant2 : Constant  Value=0.5
  Downstream (Sink) : sh_lib/Low-Pressure Blocks/Constant Head Tank  press=0 Pa  fluid_level=0 m  pipe_diam=0.02 m  loss_coeff=1.2  g=9.80665 m/s^2  volume_specify=on  volume_priority=High  volume=0 m^3  volume_nominal_specify=off  volume_nominal_unit=m^3  volume_nominal_value=1
      settings: SourceProductBaseCode=SH  InternalSimscapePortConfiguration="{\"Bottom\":[],\"Left\":[],\"Right\":[{\"id\":\"V\",\"label\":\"V\",\"type\":\"output\"},{\"id\":\"T\",\"label\":\"T\",\"type\":\"foundation.hydraulic.hydraulic\"}],\"Top\":[]}"
  Flow Divider : sh_lib/Valves/Flow Control Valves/Flow Divider  area_A=1e-4 m^2  area_B=1e-4 m^2  C_d_A=0.7  C_d_B=0.7  lam_spec=2  B_lam_A=0.999  B_lam_B=0.999  Re_cr_A=2300  Re_cr_B=2300  orifice_d=0.005 m  orifice_numb=4  C_d_or=0.65  init_A=0.0025 m  init_B=0.0025 m  leak_area=1e-9 m^2  lam_spec_or=1  B_lam_or_A=0.999  B_lam_or_B=0.999  Re_cr_or_A=10  Re_cr_or_B=10  area_sc=1.6e-4 m^2  stroke=0.005 m  spring_rate=1e3 N/m  damping=150 N/(m/s)  stop_coefficient=1e12 s*N/m^2
      settings: SourceProductBaseCode=SH  InternalSimscapePortConfiguration="{\"Bottom\":[],\"Left\":[{\"id\":\"P\",\"label\":\"P\",\"type\":\"foundation.hydraulic.hydraulic\"}],\"Right\":[{\"id\":\"A\",\"label\":\"A\",\"type\":\"foundation.hydraulic.hydraulic\"},{\"id\":\"B\",\"label\":\"B\",\"type\":\"foundation.hydraulic.hydraulic\"}],\"Top\":[]}"
  Flow Divider1 : sh_lib/Valves/Flow Control Valves/Flow Divider  area_A=1e-4 m^2  area_B=1e-4 m^2  C_d_A=0.7  C_d_B=0.7  lam_spec=2  B_lam_A=0.999  B_lam_B=0.999  Re_cr_A=2300  Re_cr_B=2300  orifice_d=0.005 m  orifice_numb=4  C_d_or=0.65  init_A=0.0025 m  init_B=0.0025 m  leak_area=1e-9 m^2  lam_spec_or=1  B_lam_or_A=0.999  B_lam_or_B=0.999  Re_cr_or_A=10  Re_cr_or_B=10  area_sc=1.6e-4 m^2  stroke=0.005 m  spring_rate=1e3 N/m  damping=150 N/(m/s)  stop_coefficient=1e12 s*N/m^2
      settings: SourceProductBaseCode=SH  InternalSimscapePortConfiguration="{\"Bottom\":[],\"Left\":[{\"id\":\"P\",\"label\":\"P\",\"type\":\"foundation.hydraulic.hydraulic\"}],\"Right\":[{\"id\":\"A\",\"label\":\"A\",\"type\":\"foundation.hydraulic.hydraulic\"},{\"id\":\"B\",\"label\":\"B\",\"type\":\"foundation.hydraulic.hydraulic\"}],\"Top\":[]}"
  Poppet Valve1 : sh_lib/Valves/Flow Control Valves/Poppet Valve  d_stem=0.01 m  cone_angle=120 deg  x_0=0 m  C_d=0.65  A_leak=1e-12 m^2  lam_spec=1  B_lam=0.999  Re_cr=10
      settings: SourceProductBaseCode=SH  InternalSimscapePortConfiguration="{\"Bottom\":[],\"Left\":[{\"id\":\"S\",\"label\":\"S\",\"type\":\"input\"},{\"id\":\"A\",\"label\":\"A\",\"type\":\"foundation.hydraulic.hydraulic\"}],\"Right\":[{\"id\":\"B\",\"label\":\"B\",\"type\":\"foundation.hydraulic.hydraulic\"}],\"Top\":[]}"
  Product : sh_lib/Local Hydraulic Resistances/Local Resistance  area=1e-4 m^2  mdl_type=1  kp_d=2  kp_r=2  lam_spec=2  B_lam=0.999  Re_cr=2300  Re_vec=[-4000, -3000, -2000, -1000, -500, -200, -100, -50, -40, -30, -20, -15, -10, 10, 20, 30, 40, 50, 100, 200, 500, 1000, 2000, 4000, 5000, 10000]  loss_coeff_vec=[.25, .3, .65, .9, .65, .75, .9, 1.15, 1.35, 1.65, 2.3, 2.8, 3.1, 5, 2.7, 1.8, 1.46, 1.3, .9, .65, .42, .3, .2, .4, .42, .25]  interp_method=2  extrap_method=2  flow_rate_threshold=1e-6 m^3/s  flow_rate_specify=off  flow_rate_priority=None  flow_rate=0 m^3/s  flow_rate_nominal_specify=off  flow_rate_nominal_unit=m^3/s  flow_rate_nominal_value=1  pressure_drop_specify=on  pressure_drop_priority=None  pressure_drop=10 psi  pressure_drop_nominal_specify=off  pressure_drop_nominal_unit=Pa  pressure_drop_nominal_value=1
      settings: SourceProductBaseCode=SH  InternalSimscapePortConfiguration="{\"Bottom\":[],\"Left\":[{\"id\":\"A\",\"label\":\"A\",\"type\":\"foundation.hydraulic.hydraulic\"}],\"Right\":[{\"id\":\"B\",\"label\":\"B\",\"type\":\"foundation.hydraulic.hydraulic\"}],\"Top\":[]}"
  Retentate : sh_lib/Local Hydraulic Resistances/Local Resistance  area=1e-4 m^2  mdl_type=1  kp_d=2  kp_r=2  lam_spec=2  B_lam=0.999  Re_cr=2300  Re_vec=[-4000, -3000, -2000, -1000, -500, -200, -100, -50, -40, -30, -20, -15, -10, 10, 20, 30, 40, 50, 100, 200, 500, 1000, 2000, 4000, 5000, 10000]  loss_coeff_vec=[.25, .3, .65, .9, .65, .75, .9, 1.15, 1.35, 1.65, 2.3, 2.8, 3.1, 5, 2.7, 1.8, 1.46, 1.3, .9, .65, .42, .3, .2, .4, .42, .25]  interp_method=2  extrap_method=2  flow_rate_threshold=1e-6 m^3/s  flow_rate_specify=off  flow_rate_priority=None  flow_rate=0 m^3/s  flow_rate_nominal_specify=off  flow_rate_nominal_unit=m^3/s  flow_rate_nominal_value=1  pressure_drop_specify=on  pressure_drop_priority=None  pressure_drop=10 psi  pressure_drop_nominal_specify=off  pressure_drop_nominal_unit=Pa  pressure_drop_nominal_value=1
      settings: SourceProductBaseCode=SH  InternalSimscapePortConfiguration="{\"Bottom\":[],\"Left\":[{\"id\":\"A\",\"label\":\"A\",\"type\":\"foundation.hydraulic.hydraulic\"}],\"Right\":[{\"id\":\"B\",\"label\":\"B\",\"type\":\"foundation.hydraulic.hydraulic\"}],\"Top\":[]}"
  Simulink-PS Converter1 : nesl_utility/Simulink-PS Converter  PhysicalDomain=network_engine_domain  SubClassName=ps_input  LeftPortType=input  RightPortType=output  PseudoPeriodic=off  Frequencies=[]  NoiseDistribution=none  NoiseParameters=[]  Unit=1  AffineConversion=off  FilteringAndDerivatives=zero  SimscapeFilterOrder=1  InputFilterTimeConstant=.001  UdotUserProvided=0
  Simulink-PS Converter2 : nesl_utility/Simulink-PS Converter  PhysicalDomain=network_engine_domain  SubClassName=ps_input  LeftPortType=input  RightPortType=output  PseudoPeriodic=off  Frequencies=[]  NoiseDistribution=none  NoiseParameters=[]  Unit=1  AffineConversion=off  FilteringAndDerivatives=zero  SimscapeFilterOrder=1  InputFilterTimeConstant=.001  UdotUserProvided=0
  IN : PMIOPort  Side=Left
  OUT : PMIOPort  Port=2  Side=Right
  wires:
  Constant/1 -> Simulink-PS Converter1/1
  Constant1/1 -> Centrifugal Pump3/1(f)
  Constant2/1 -> Simulink-PS Converter2/1
  connections:
  Retentate/LConn1 -- Flow Divider/RConn1
  Flow Divider/RConn2 -- Product/LConn1
  Flow Divider/LConn1 -- Flow Divider1/RConn2
  Flow Divider1/RConn1 -- Bypass Valve/LConn2
  Centrifugal Pump3/RConn1 -- Flow Divider1/LConn1
  IN/RConn1 -- Centrifugal Pump3/LConn1
  Simulink-PS Converter1/RConn1 -- Bypass Valve/LConn1
  Bypass Valve/RConn1 -- Bypass/LConn1
  Retentate/RConn1 -- Check Valve/RConn1
  Poppet Valve1/LConn1 -- Simulink-PS Converter2/RConn1
  Poppet Valve1/RConn1 -- Downstream (Sink)/RConn2
  Poppet Valve1/LConn2 -- Check Valve/LConn1
  OUT/RConn1 -- Product/RConn1 -- Bypass/RConn1

== system RO_Plantsimscape/F_GAC1 ==
  Hydraulic Flow Rate Sensor : fl_lib/Hydraulic/Hydraulic Sensors/Hydraulic Flow Rate Sensor
  PS-Simulink Converter3 : nesl_utility/PS-Simulink Converter  PhysicalDomain=network_engine_domain  SubClassName=ps_output  LeftPortType=input  RightPortType=output  PseudoPeriodic=off  Frequencies=[]  Unit=1  AffineConversion=off
  Resistive Pipe LP : sh_lib/Low-Pressure Blocks/Resistive Pipe LP  cs_type=1  d_in=10 in  area=1e-4 m^2  D_h=1.12e-2 m  s_factor=64  length=5 m  length_ad=1 m  roughness=15e-6 m  Re_lam=2000  Re_turb=4000  elevation_A=0 m  elevation_B=0 m  g=9.80665 m/s^2  pressure_drop_specify=off  pressure_drop_priority=None  pressure_drop=0 Pa  pressure_drop_nominal_specify=off  pressure_drop_nominal_unit=Pa  pressure_drop_nominal_value=1  flow_rate_specify=off  flow_rate_priority=None  flow_rate=0 m^3/s  flow_rate_nominal_specify=off  flow_rate_nominal_unit=m^3/s  flow_rate_nominal_value=1
      settings: SourceProductBaseCode=SH  InternalSimscapePortConfiguration="{\"Bottom\":[],\"Left\":[{\"id\":\"A\",\"label\":\"A\",\"type\":\"foundation.hydraulic.hydraulic\"}],\"Right\":[{\"id\":\"B\",\"label\":\"B\",\"type\":\"foundation.hydraulic.hydraulic\"}],\"Top\":[]}"
  Scope3 : Scope
  IN : PMIOPort  Side=Left
  OUT : PMIOPort  Port=2  Side=Right
  wires:
  PS-Simulink Converter3/1 -> Scope3/1
  connections:
  Resistive Pipe LP/LConn1 -- IN/RConn1
  Hydraulic Flow Rate Sensor/RConn2 -- OUT/RConn1
  Hydraulic Flow Rate Sensor/RConn1 -- PS-Simulink Converter3/LConn1
  Resistive Pipe LP/RConn1 -- Hydraulic Flow Rate Sensor/LConn1

== system RO_Plantsimscape/P1 ==
  Hydraulic Flow Rate Sensor1 : fl_lib/Hydraulic/Hydraulic Sensors/Hydraulic Flow Rate Sensor
  Resistive Pipe LP : sh_lib/Low-Pressure Blocks/Resistive Pipe LP  cs_type=1  d_in=10 in  area=1e-4 m^2  D_h=1.12e-2 m  s_factor=64  length=15 m  length_ad=1 m  roughness=0.061 m  Re_lam=2000  Re_turb=4000  elevation_A=0 m  elevation_B=10 m  g=9.81 m/s^2  pressure_drop_specify=off  pressure_drop_priority=None  pressure_drop=0 Pa  pressure_drop_nominal_specify=off  pressure_drop_nominal_unit=Pa  pressure_drop_nominal_value=1  flow_rate_specify=off  flow_rate_priority=None  flow_rate=0 m^3/s  flow_rate_nominal_specify=off  flow_rate_nominal_unit=m^3/s  flow_rate_nominal_value=1
      settings: SourceProductBaseCode=SH  InternalSimscapePortConfiguration="{\"Bottom\":[],\"Left\":[{\"id\":\"A\",\"label\":\"A\",\"type\":\"foundation.hydraulic.hydraulic\"}],\"Right\":[{\"id\":\"B\",\"label\":\"B\",\"type\":\"foundation.hydraulic.hydraulic\"}],\"Top\":[]}"
  Resistive Pipe LP1 : sh_lib/Low-Pressure Blocks/Resistive Pipe LP  cs_type=1  d_in=10 in  area=1e-4 m^2  D_h=1.12e-2 m  s_factor=64  length=10 m  length_ad=1 m  roughness=0.061 m  Re_lam=2000  Re_turb=4000  elevation_A=0 m  elevation_B=0 m  g=9.81 m/s^2  pressure_drop_specify=off  pressure_drop_priority=None  pressure_drop=0 Pa  pressure_drop_nominal_specify=off  pressure_drop_nominal_unit=Pa  pressure_drop_nominal_value=1  flow_rate_specify=off  flow_rate_priority=None  flow_rate=0 m^3/s  flow_rate_nominal_specify=off  flow_rate_nominal_unit=m^3/s  flow_rate_nominal_value=1
      settings: SourceProductBaseCode=SH  InternalSimscapePortConfiguration="{\"Bottom\":[],\"Left\":[{\"id\":\"A\",\"label\":\"A\",\"type\":\"foundation.hydraulic.hydraulic\"}],\"Right\":[{\"id\":\"B\",\"label\":\"B\",\"type\":\"foundation.hydraulic.hydraulic\"}],\"Top\":[]}"
  Resistive Pipe LP2 : sh_lib/Low-Pressure Blocks/Resistive Pipe LP  cs_type=1  d_in=10 in  area=1e-4 m^2  D_h=1.12e-2 m  s_factor=64  length=60 m  length_ad=1 m  roughness=0.061 m  Re_lam=2000  Re_turb=4000  elevation_A=0 m  elevation_B=10 m  g=9.81 m/s^2  pressure_drop_specify=off  pressure_drop_priority=None  pressure_drop=0 Pa  pressure_drop_nominal_specify=off  pressure_drop_nominal_unit=Pa  pressure_drop_nominal_value=1  flow_rate_specify=off  flow_rate_priority=None  flow_rate=0 m^3/s  flow_rate_nominal_specify=off  flow_rate_nominal_unit=m^3/s  flow_rate_nominal_value=1
      settings: SourceProductBaseCode=SH  InternalSimscapePortConfiguration="{\"Bottom\":[],\"Left\":[{\"id\":\"A\",\"label\":\"A\",\"type\":\"foundation.hydraulic.hydraulic\"}],\"Right\":[{\"id\":\"B\",\"label\":\"B\",\"type\":\"foundation.hydraulic.hydraulic\"}],\"Top\":[]}"
  T-junction : sh_lib/Local Hydraulic Resistances/T-junction  main_diam=0.01 m  branch_diam=0.01 m  kp_ab=1.12  kp_ba=1.12  kp_aa1=1.36  kp_a1a=1.65  kp_a1b=1.6  kp_ba1=1.8  lam_spec=1  B_lam=0.999  Re_cr=120
      settings: SourceProductBaseCode=SH  InternalSimscapePortConfiguration="{\"Bottom\":[],\"Left\":[{\"id\":\"A\",\"label\":\"A\",\"type\":\"foundation.hydraulic.hydraulic\"},{\"id\":\"A1\",\"label\":\"A1\",\"type\":\"foundation.hydraulic.hydraulic\"}],\"Right\":[{\"id\":\"B\",\"label\":\"B\",\"type\":\"foundation.hydraulic.hydraulic\"}],\"Top\":[]}"
  IN : PMIOPort  Side=Left
  OUT : PMIOPort  Port=2  Side=Right
  OUT1 : PMIOPort  Port=3  Side=Right
  connections:
  Hydraulic Flow Rate Sensor1/RConn2 -- OUT/RConn1
  Resistive Pipe LP1/LConn1 -- IN/RConn1
  Resistive Pipe LP/RConn1 -- Hydraulic Flow Rate Sensor1/LConn1
  Resistive Pipe LP/LConn1 -- T-junction/RConn1
  T-junction/LConn1 -- Resistive Pipe LP1/RConn1
  Resistive Pipe LP2/RConn1 -- OUT1/RConn1
  Resistive Pipe LP2/LConn1 -- T-junction/LConn2

== system RO_Plantsimscape/P10 ==
  Hydraulic Flow Rate Sensor1 : fl_lib/Hydraulic/Hydraulic Sensors/Hydraulic Flow Rate Sensor
  Resistive Pipe LP1 : sh_lib/Low-Pressure Blocks/Resistive Pipe LP  cs_type=1  d_in=4 in  area=1e-4 m^2  D_h=1.12e-2 m  s_factor=64  length=30 m  length_ad=1 m  roughness=0.061 m  Re_lam=2000  Re_turb=4000  elevation_A=0 m  elevation_B=0 m  g=9.81 m/s^2  pressure_drop_specify=off  pressure_drop_priority=None  pressure_drop=0 Pa  pressure_drop_nominal_specify=off  pressure_drop_nominal_unit=Pa  pressure_drop_nominal_value=1  flow_rate_specify=off  flow_rate_priority=None  flow_rate=0 m^3/s  flow_rate_nominal_specify=off  flow_rate_nominal_unit=m^3/s  flow_rate_nominal_value=1
      settings: SourceProductBaseCode=SH  InternalSimscapePortConfiguration="{\"Bottom\":[],\"Left\":[{\"id\":\"A\",\"label\":\"A\",\"type\":\"foundation.hydraulic.hydraulic\"}],\"Right\":[{\"id\":\"B\",\"label\":\"B\",\"type\":\"foundation.hydraulic.hydraulic\"}],\"Top\":[]}"
  IN : PMIOPort  Side=Left
  OUT : PMIOPort  Port=2  Side=Right
  connections:
  Resistive Pipe LP1/RConn1 -- Hydraulic Flow Rate Sensor1/LConn1
  Hydraulic Flow Rate Sensor1/RConn2 -- OUT/RConn1
  Resistive Pipe LP1/LConn1 -- IN/RConn1

== system RO_Plantsimscape/P11 ==
  Hydraulic Flow Rate Sensor1 : fl_lib/Hydraulic/Hydraulic Sensors/Hydraulic Flow Rate Sensor
  Resistive Pipe LP1 : sh_lib/Low-Pressure Blocks/Resistive Pipe LP  cs_type=1  d_in=10 in  area=1e-4 m^2  D_h=1.12e-2 m  s_factor=64  length=15 m  length_ad=1 m  roughness=0.061 m  Re_lam=2000  Re_turb=4000  elevation_A=0 m  elevation_B=0 m  g=9.81 m/s^2  pressure_drop_specify=off  pressure_drop_priority=None  pressure_drop=0 Pa  pressure_drop_nominal_specify=off  pressure_drop_nominal_unit=Pa  pressure_drop_nominal_value=1  flow_rate_specify=off  flow_rate_priority=None  flow_rate=0 m^3/s  flow_rate_nominal_specify=off  flow_rate_nominal_unit=m^3/s  flow_rate_nominal_value=1
      settings: SourceProductBaseCode=SH  InternalSimscapePortConfiguration="{\"Bottom\":[],\"Left\":[{\"id\":\"A\",\"label\":\"A\",\"type\":\"foundation.hydraulic.hydraulic\"}],\"Right\":[{\"id\":\"B\",\"label\":\"B\",\"type\":\"foundation.hydraulic.hydraulic\"}],\"Top\":[]}"
  IN : PMIOPort  Side=Left
  OUT : PMIOPort  Port=2  Side=Right
  connections:
  Resistive Pipe LP1/RConn1 -- Hydraulic Flow Rate Sensor1/LConn1
  Hydraulic Flow Rate Sensor1/RConn2 -- OUT/RConn1
  Resistive Pipe LP1/LConn1 -- IN/RConn1
